simulink model "sl_sea"  (R2015b)
settings: Solver=VariableStepAuto  StartTime=0.0  StopTime=5  RelTol=1e-3
libraries: simulink x1
settings Model: Creator=corkep  LastModifiedBy=corkep
settings DataIOCC: SaveFormat=Array  ReturnWorkspaceOutputs=on  TimeSaveName=t  OutputSaveName=y

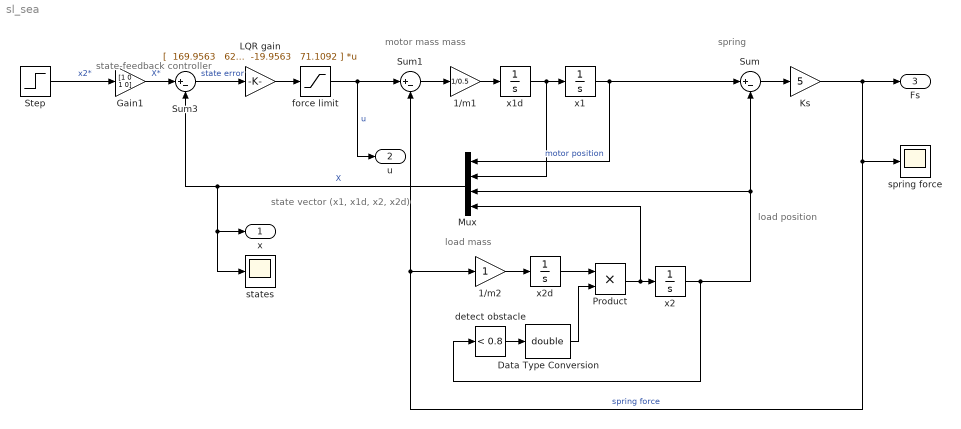
== system sl_sea ==
  note: spring
  note: state vector (x1, x1d, x2, x2d)
  note: load position
  note: motor mass mass
  note: load mass
  note: state-feedback controller
  1/m1 : Gain  Gain=1/0.5
  1/m2 : Gain
  Data Type Conversion : DataTypeConversion  OutDataTypeStr=double
  Gain1 : Gain  Gain=[1 0 1 0]
  Ks : Gain  Gain=5
  LQR gain : Gain  Gain=|  Multiplication=Matrix(K*u)
      | [  169.9563   62.9010  -19.9563   71.1092
      | ]
  Mux : Mux
  Product : Product
  Step : Step  SampleTime=0
  Sum : Sum  Inputs=|+-
  Sum1 : Sum  Inputs=|+-
  Sum3 : Sum  Inputs=|+-
  detect obstacle : simulink/Logic and Bit Operations/Compare To Constant  relop=<  const=0.8  OutDataTypeStr=boolean
  force limit : Saturate  UpperLimit=2  LowerLimit=-2
  spring force : Scope
  states : Scope
  x1 : Integrator
  x1d : Integrator
  x2 : Integrator
  x2d : Integrator
  x : Outport
  u : Outport  Port=2
  Fs : Outport  Port=3
  wires:
  x1/1 -> Mux/1, Sum/1  "motor position"
  Sum/1 -> Ks/1
  x2d/1 -> Product/1
  Step/1 -> Gain1/1  "x2*"
  x1d/1 -> Mux/2, x1/1
  Sum1/1 -> 1/m1/1
  Sum3/1 -> LQR gain/1  "state error"
  LQR gain/1 -> force limit/1
  1/m1/1 -> x1d/1
  1/m2/1 -> x2d/1
  Gain1/1 -> Sum3/1  "X*"
  Mux/1 -> x/1, states/1, Sum3/2  "X"
  Ks/1 -> Sum1/2, 1/m2/1, spring force/1, Fs/1  "spring force"
  Product/1 -> Mux/4, x2/1
  Data Type Conversion/1 -> Product/2
  detect obstacle/1 -> Data Type Conversion/1
  force limit/1 -> u/1, Sum1/1  "u"
  x2/1 -> detect obstacle/1, Mux/3, Sum/2
